simulink model "Day_08_Sliding_Mode_Control"  (R2024a)
settings: Solver=daessc  StartTime=0.0  StopTime=3  FixedStep=0.001  RelTol=1e-3
values from neighbouring files (symbols this model uses):
  C_theta = 3    [Day_08.m]
  C_x = 1    [Day_08.m]
  D0 = 2700    [Day_08.m]
  D1 = 2700    [Day_08.m]
  epsilon = 0.5    [Day_08.m]
  K = 100    [Day_08.m]
  L0 = 0.01    [Day_08.m]
  L1 = 0.14    [Day_08.m]
  lambda = 1    [Day_08.m]
  limit = .45    (= 0.45)    [Day_08.m]
  m = 3    [Day_08.m]
  M0 = L0*W0*T0*D0    (= 0.0027)    [Day_08.m]
  M1 = L1*W1*T1*D1    (= 0.0378)    [Day_08.m]
  T0 = 0.01    [Day_08.m]
  T1 = 0.01    [Day_08.m]
  W0 = 0.01    [Day_08.m]
  W1 = 0.01    [Day_08.m]
  x1_d = 0    [Day_08.m]
  x2_d = 0    [Day_08.m]
  x3_d = 0    [Day_08.m]
  x4_d = 0    [Day_08.m]
undefined symbols (not defined in the file or in its folder): X, Y, Z
libraries: sm_lib x14, nesl_utility x7
settings Model: Creator=mingeun  LastModifiedBy=mingeun
settings SolverCC: ZeroCrossAlgorithm=Adaptive
settings DataIOCC: ReturnWorkspaceOutputs=off
settings OptimizationCC: BlockReduction=off  DefaultParameterBehavior=Inlined  BufferReuse=off
settings DebuggingCC: IgnoredZcDiagnostic=none

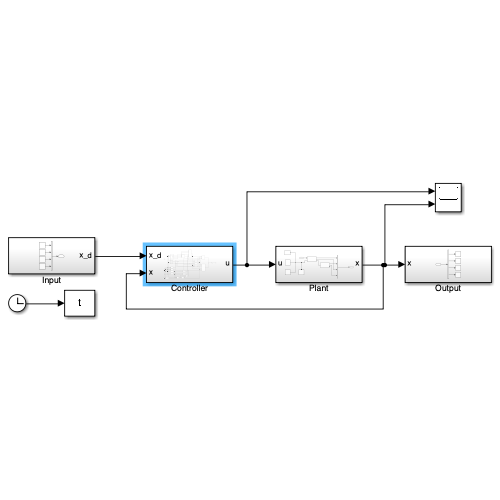
[thumbnail: Simulink's stored preview of the top-level diagram]
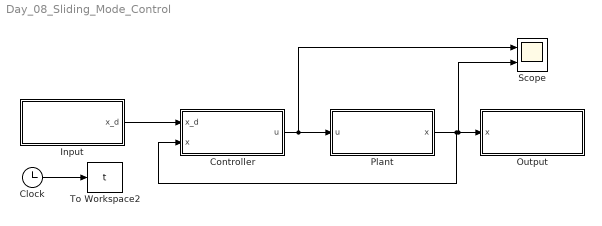
== system Day_08_Sliding_Mode_Control ==
  Clock : Clock
  Controller : Subsystem
  Input : Subsystem
  Output : Subsystem
  Plant : Subsystem
  Scope : Scope  NumInputPorts=2
  To Workspace2 : ToWorkspace  VariableName=t  SampleTime=-1
  wires:
  Clock/1 -> To Workspace2/1
  Input/1(x_d) -> Controller/1(x_d)
  Controller/1(u) -> Scope/1, Plant/1(u)
  Plant/1(x) -> Scope/2, Output/1(x), Controller/2(x)

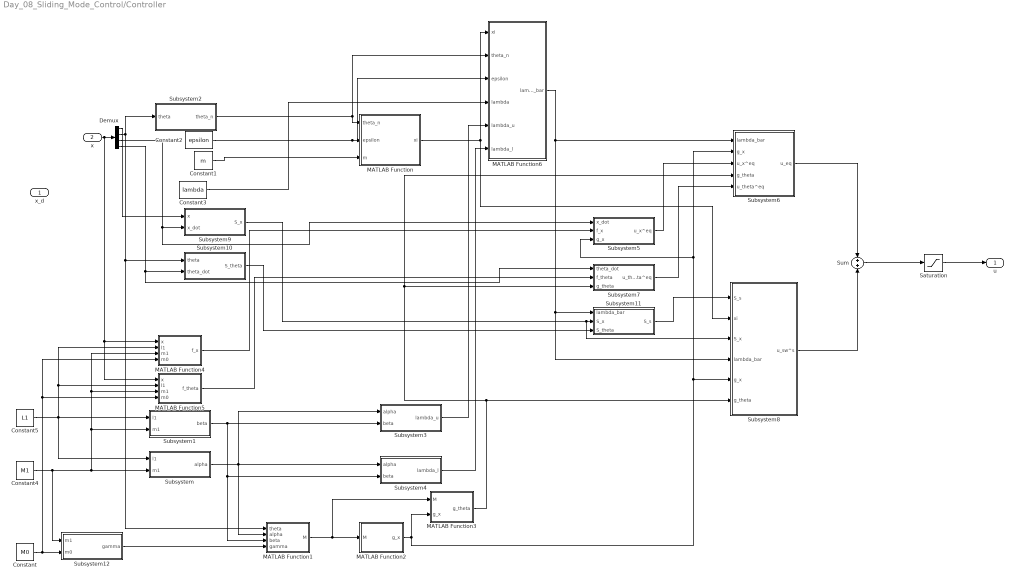
== system Day_08_Sliding_Mode_Control/Controller ==
  x_d : Inport
  x : Inport  Port=2
  Constant : Constant  Value=M0
  Constant1 : Constant  Value=m
  Constant2 : Constant  Value=epsilon
  Constant3 : Constant  Value=lambda
  Constant4 : Constant  Value=M1
  Constant5 : Constant  Value=L1
  Demux : Demux
  MATLAB Function : MATLAB Function  TreatAsAtomicUnit=on
  MATLAB Function1 : MATLAB Function  TreatAsAtomicUnit=on
  MATLAB Function2 : MATLAB Function  TreatAsAtomicUnit=on
  MATLAB Function3 : MATLAB Function  TreatAsAtomicUnit=on
  MATLAB Function4 : MATLAB Function  TreatAsAtomicUnit=on
  MATLAB Function5 : MATLAB Function  TreatAsAtomicUnit=on
  MATLAB Function6 : MATLAB Function  TreatAsAtomicUnit=on
  Saturation : Saturate  UpperLimit=limit  LowerLimit=-limit
  Subsystem : Subsystem
  Subsystem1 : Subsystem
  Subsystem10 : Subsystem
  Subsystem11 : Subsystem
  Subsystem12 : Subsystem
  Subsystem2 : Subsystem
  Subsystem3 : Subsystem
  Subsystem4 : Subsystem
  Subsystem5 : Subsystem
  Subsystem6 : Subsystem
  Subsystem7 : Subsystem
  Subsystem8 : Subsystem
  Subsystem9 : Subsystem
  Sum : Sum  Inputs=+|+
  u : Outport
  wires:
  Saturation/1 -> u/1
  x/1 -> Demux/1, MATLAB Function5/1(x), MATLAB Function4/1(x)
  Demux/2 -> Subsystem2/1(theta), Subsystem10/1(theta), MATLAB Function1/1(theta)
  Constant1/1 -> MATLAB Function/3(m)
  Constant2/1 -> MATLAB Function6/3(epsilon), MATLAB Function/2(epsilon)
  Constant5/1 -> Subsystem1/1(l1), Subsystem/1(l1), MATLAB Function5/2(l1), MATLAB Function4/2(l1)
  Constant4/1 -> Subsystem1/2(m1), MATLAB Function5/3(m1), MATLAB Function4/3(m1), Subsystem/2(m1), Subsystem12/1(m1)
  Subsystem/1(alpha) -> MATLAB Function1/2(alpha), Subsystem3/1(alpha), Subsystem4/1(alpha)
  Subsystem1/1(beta) -> MATLAB Function1/3(beta), Subsystem4/2(beta), Subsystem3/2(beta)
  Constant/1 -> MATLAB Function5/4(m0), MATLAB Function4/4(m0), Subsystem12/2(m0)
  MATLAB Function1/1(M) -> MATLAB Function3/1(M), MATLAB Function2/1(M)
  MATLAB Function2/1(g_x) -> Subsystem8/5(g_x), Subsystem6/2(g_x), Subsystem5/3(g_x), MATLAB Function3/2(g_x)
  Subsystem2/1(theta_n) -> MATLAB Function6/2(theta_n), MATLAB Function/1(theta_n)
  Constant3/1 -> MATLAB Function6/4(lambda)
  Subsystem3/1(lambda_u) -> MATLAB Function6/5(lambda_u)
  Subsystem4/1(lambda_l) -> MATLAB Function6/6(lambda_l)
  MATLAB Function3/1(g_theta) -> Subsystem7/3(g_theta), Subsystem6/4(g_theta), Subsystem8/6(g_theta)
  Demux/3 -> Subsystem9/2(x_dot), Subsystem5/1(x_dot)
  Demux/4 -> Subsystem7/1(theta_dot), Subsystem10/2(theta_dot)
  MATLAB Function4/1(f_x) -> Subsystem5/2(f_x)
  MATLAB Function5/1(f_theta) -> Subsystem7/2(f_theta)
  Subsystem7/1(u_theta^eq) -> Subsystem6/5(u_theta^eq)
  Subsystem5/1(u_x^eq) -> Subsystem6/3(u_x^eq)
  Demux/1 -> Subsystem9/1(x)
  Subsystem9/1(S_x) -> Subsystem8/3(S_x), Subsystem11/2(S_x)
  Subsystem10/1(S_theta) -> Subsystem11/3(S_theta)
  Subsystem11/1(S_s) -> Subsystem8/1(S_s)
  MATLAB Function/1(xi) -> MATLAB Function6/1(xi), Subsystem8/2(xi)
  MATLAB Function6/1(lambda_bar) -> Subsystem8/4(lambda_bar), Subsystem11/1(lambda_bar), Subsystem6/1(lambda_bar)
  Subsystem6/1(u_eq) -> Sum/1
  Subsystem8/1(u_sw^s) -> Sum/2
  Sum/1 -> Saturation/1
  Subsystem12/1(gamma) -> MATLAB Function1/4(gamma)

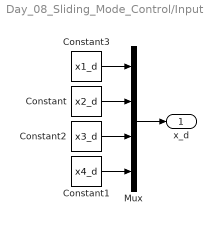
== system Day_08_Sliding_Mode_Control/Input ==
  Constant : Constant  Value=x2_d
  Constant1 : Constant  Value=x4_d
  Constant2 : Constant  Value=x3_d
  Constant3 : Constant  Value=x1_d
  Mux : Mux
  x_d : Outport
  wires:
  Mux/1 -> x_d/1
  Constant1/1 -> Mux/4
  Constant2/1 -> Mux/3
  Constant/1 -> Mux/2
  Constant3/1 -> Mux/1

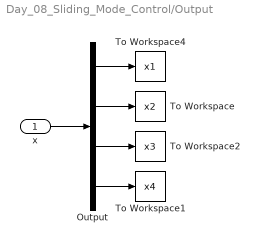
== system Day_08_Sliding_Mode_Control/Output ==
  x : Inport
  Output : Demux
  To Workspace : ToWorkspace  VariableName=x2  SampleTime=-1
  To Workspace1 : ToWorkspace  VariableName=x4  SampleTime=-1
  To Workspace2 : ToWorkspace  VariableName=x3  SampleTime=-1
  To Workspace4 : ToWorkspace  VariableName=x1  SampleTime=-1
  wires:
  Output/3 -> To Workspace2/1
  Output/4 -> To Workspace1/1
  Output/2 -> To Workspace/1
  Output/1 -> To Workspace4/1
  x/1 -> Output/1

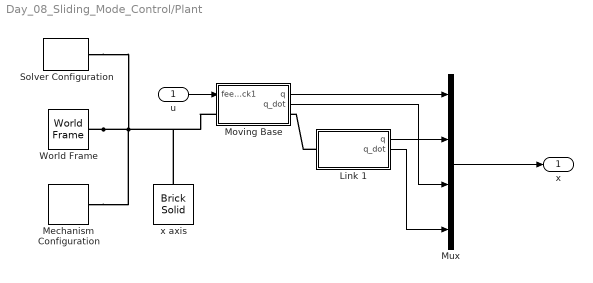
== system Day_08_Sliding_Mode_Control/Plant ==
  u : Inport
  Link 1 : Subsystem  mask{L=L1*100, W=W1*100, H=T1*100, rho=D1, rgb=[0.25 0.40 0.70], angle=150, F=0}
      mask prompts: L "Length (cm)"; W "Width (cm)"; H "Thickness (cm)"; rho "Density (kg/m^3)"; rgb "Color [R G B]"; angle "Initial Angle (degree)"; F "Disturbance [N]"
  Mechanism Configuration : sm_lib/Utilities/Mechanism Configuration  UniformGravity=Constant  GravityVector=[0 0 -9.80665]  GravityVectorUnits=m/s^2  LinearizationDelta=0.001  JointModeTransitionNonlinearIterations=2
  Moving Base : Subsystem  mask{L=L0*100, W=W0*100, H=T0*100, rho=D0, RGB=[0.8 0.45 0.0]}
      mask prompts: L "Length (cm)"; W "Width (cm)"; H "Thickness (cm)"; rho "Density (kg/m^3)"; RGB "Color [R G B]"
  Mux : Mux
  Solver Configuration : nesl_utility/Solver Configuration  PhysicalDomain=network_engine_domain  SubClassName=solver  LeftPortType=input  RightPortType=generic  Tones=[]  Harmonics=[]  SimulateNoise=off  Profile=off  UseLocalSampling=off  EnableSwitchedLinearOptims=on  FrequencyDomain=off  UseCCode=off  RelTol=0.001  AbsTol=0.001  MinStep=1e-09  ToWorkspace=off  RevertToSquareIcSolve=off  NumHomotopyIterations=100  PhasorMode=off  PhasorModeNumHarmonics=1  ConsistencySolver=NEWTON_XTOL_AFTER_FTOL  IndexReductionMethod=DerivativeReplacement  DoDC=off  ResidualTolerance=1e-09  ConsistencyTolSource=GLOBAL  ConsistencyAbsTol=0.001  ConsistencyRelTol=0.001  ConsistencyTolFactor=0.001  UseLocalSolver=off  LocalSolverChoice=NE_BACKWARD_EULER_ADVANCER  ResolveIndetEquations=on  FunctionEvalNumThread=1  LocalSolverSampleTime=0.001  DoFixedCost=off  MaxNonlinIter=3  MaxModeIter=2  ComputeImpulses=off  ImpulseIterations=2  LinearAlgebra=auto  LinearAlgebraNumThread=0  EquationFormulation=NE_TIME_EF  DelaysMemoryBudget=1024  AutomaticFiltering=on  FilteringTimeConstant=0.001  PartitionStorageMethod=AS_NEEDED  PartitionMemoryBudget=1024  PartitionMethod=ROBUST  MultibodyUseLocalSolver=off  MultibodyLocalSolverChoice=ODE1  MultibodyLocalSolverSampleTime=0.001
  World Frame : sm_lib/Frames and Transforms/World Frame
  x axis : sm_lib/Body Elements/Brick Solid  BrickDimensions=[1000 1 1]  BrickDimensionsUnits=mm  ExportEntireGeometry=off  InertiaType=CalculateFromGeometry  BasedOnType=Density  Density=1000  DensityUnits=kg/m^3  Mass=1  MassUnits=kg  CenterOfMass=[0 0 0]  CenterOfMassUnits=m  MomentsOfInertia=[1 1 1]  MomentsOfInertiaUnits=kg*m^2  ProductsOfInertia=[0 0 0]  ProductsOfInertiaUnits=kg*m^2  GraphicType=FromGeometry  MarkerShape=Sphere  MarkerSize=10  GraphicVisPropType=SimpleVisualProperties  GraphicDiffuseColor=[0.0 0.0 0.0]  GraphicOpacity=1  GraphicSpecularColor=[0.5 0.5 0.5 1.0]  GraphicAmbientColor=[0.15 0.15 0.15 1.0]  GraphicEmissiveColor=[0.0 0.0 0.0 1.0]  GraphicShininess=75  DoExposeReferenceFrame=on  SerializedFrames=<Frames/>
  x : Outport
  wires:
  Moving Base/1(q) -> Mux/1
  Link 1/1(q) -> Mux/2
  u/1 -> Moving Base/1(feedback1)
  Link 1/2(q_dot) -> Mux/4
  Moving Base/2(q_dot) -> Mux/3
  Mux/1 -> x/1
  connections:
  World Frame/RConn1 -- Solver Configuration/RConn1 -- Moving Base/LConn1 -- x axis/RConn1 -- Mechanism Configuration/RConn1
  Link 1/LConn1 -- Moving Base/RConn1

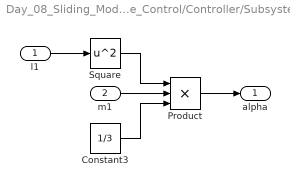
== system Day_08_Sliding_Mode_Control/Controller/Subsystem ==
  l1 : Inport
  m1 : Inport  Port=2
  Constant3 : Constant  Value=1/3
  Product : Product  Inputs=3
  Square : Math  Operator=square
  alpha : Outport
  wires:
  Product/1 -> alpha/1
  m1/1 -> Product/2
  Constant3/1 -> Product/3
  Square/1 -> Product/1
  l1/1 -> Square/1

== system Day_08_Sliding_Mode_Control/Controller/Subsystem1 ==
  l1 : Inport
  m1 : Inport  Port=2
  Constant7 : Constant  Value=1/2
  Product1 : Product  Inputs=3
  beta : Outport
  wires:
  Constant7/1 -> Product1/3
  Product1/1 -> beta/1
  l1/1 -> Product1/1
  m1/1 -> Product1/2

== system Day_08_Sliding_Mode_Control/Controller/Subsystem10 ==
  theta : Inport
  theta_dot : Inport  Port=2
  Gain : Gain  Gain=C_theta
  Sum : Sum  Inputs=|++
  S_theta : Outport
  wires:
  Sum/1 -> S_theta/1
  theta_dot/1 -> Sum/2
  Gain/1 -> Sum/1
  theta/1 -> Gain/1

== system Day_08_Sliding_Mode_Control/Controller/Subsystem11 ==
  lambda_bar : Inport
  S_x : Inport  Port=2
  S_theta : Inport  Port=3
  Product : Product
  Sum : Sum  Inputs=|++
  S_s : Outport
  wires:
  S_theta/1 -> Sum/2
  Product/1 -> Sum/1
  S_x/1 -> Product/2
  Sum/1 -> S_s/1
  lambda_bar/1 -> Product/1

== system Day_08_Sliding_Mode_Control/Controller/Subsystem12 ==
  m1 : Inport
  m0 : Inport  Port=2
  Sum : Sum  Inputs=|++
  gamma : Outport
  wires:
  Sum/1 -> gamma/1
  m0/1 -> Sum/2
  m1/1 -> Sum/1

== system Day_08_Sliding_Mode_Control/Controller/Subsystem2 ==
  theta : Inport
  Abs : Abs  SaturateOnIntegerOverflow=off
  Constant : Constant  Value=pi/2
  Sum : Sum  Inputs=|+-
  theta_n : Outport
  wires:
  Sum/1 -> theta_n/1
  Constant/1 -> Sum/2
  Abs/1 -> Sum/1
  theta/1 -> Abs/1

== system Day_08_Sliding_Mode_Control/Controller/Subsystem3 ==
  alpha : Inport
  beta : Inport  Port=2
  Divide : Product  Inputs=/**
  theta_u^star : Constant  Value=pi/2-epsilon
  lambda_u : Outport
  wires:
  Divide/1 -> lambda_u/1
  theta_u^star/1 -> Divide/3
  beta/1 -> Divide/2
  alpha/1 -> Divide/1

== system Day_08_Sliding_Mode_Control/Controller/Subsystem4 ==
  alpha : Inport
  beta : Inport  Port=2
  Divide : Product  Inputs=/**
  theta_l^star1 : Constant  Value=pi/2+epsilon
  lambda_l : Outport
  wires:
  Divide/1 -> lambda_l/1
  beta/1 -> Divide/2
  alpha/1 -> Divide/1
  theta_l^star1/1 -> Divide/3

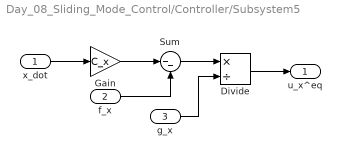
== system Day_08_Sliding_Mode_Control/Controller/Subsystem5 ==
  x_dot : Inport
  f_x : Inport  Port=2
  g_x : Inport  Port=3
  Divide : Product  Inputs=*/
  Gain : Gain  Gain=C_x
  Sum : Sum  Inputs=|--
  u_x^eq : Outport
  wires:
  Divide/1 -> u_x^eq/1
  g_x/1 -> Divide/2
  f_x/1 -> Sum/2
  Sum/1 -> Divide/1
  Gain/1 -> Sum/1
  x_dot/1 -> Gain/1

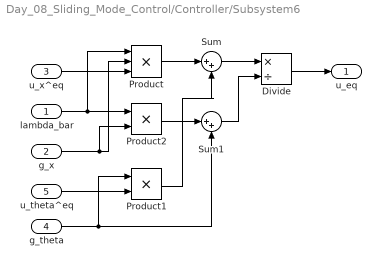
== system Day_08_Sliding_Mode_Control/Controller/Subsystem6 ==
  lambda_bar : Inport
  g_x : Inport  Port=2
  u_x^eq : Inport  Port=3
  g_theta : Inport  Port=4
  u_theta^eq : Inport  Port=5
  Divide : Product  Inputs=*/
  Product : Product  Inputs=3
  Product1 : Product
  Product2 : Product
  Sum : Sum  Inputs=|++
  Sum1 : Sum  Inputs=|++
  u_eq : Outport
  wires:
  Divide/1 -> u_eq/1
  Sum/1 -> Divide/1
  Sum1/1 -> Divide/2
  Product1/1 -> Sum/2
  Product/1 -> Sum/1
  g_theta/1 -> Product1/1, Sum1/2
  g_x/1 -> Product2/2, Product/2
  lambda_bar/1 -> Product2/1, Product/1
  u_theta^eq/1 -> Product1/2
  Product2/1 -> Sum1/1
  u_x^eq/1 -> Product/3

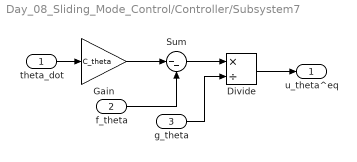
== system Day_08_Sliding_Mode_Control/Controller/Subsystem7 ==
  theta_dot : Inport
  f_theta : Inport  Port=2
  g_theta : Inport  Port=3
  Divide : Product  Inputs=*/
  Gain : Gain  Gain=C_theta
  Sum : Sum  Inputs=|--
  u_theta^eq : Outport
  wires:
  g_theta/1 -> Divide/2
  Sum/1 -> Divide/1
  Divide/1 -> u_theta^eq/1
  f_theta/1 -> Sum/2
  Gain/1 -> Sum/1
  theta_dot/1 -> Gain/1

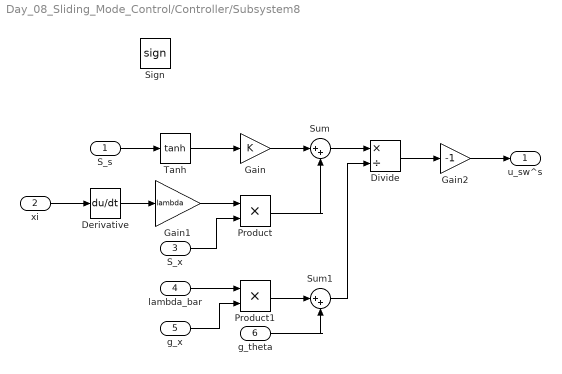
== system Day_08_Sliding_Mode_Control/Controller/Subsystem8 ==
  S_s : Inport
  xi : Inport  Port=2
  S_x : Inport  Port=3
  lambda_bar : Inport  Port=4
  g_x : Inport  Port=5
  g_theta : Inport  Port=6
  Derivative : Derivative
  Divide : Product  Inputs=*/
  Gain : Gain  Gain=K
  Gain1 : Gain  Gain=lambda
  Gain2 : Gain  Gain=-1
  Product : Product
  Product1 : Product
  Sign : Signum
  Sum : Sum  Inputs=|++
  Sum1 : Sum  Inputs=|++
  Tanh : Trigonometry  Operator=tanh
  u_sw^s : Outport
  wires:
  Gain2/1 -> u_sw^s/1
  Sum1/1 -> Divide/2
  Sum/1 -> Divide/1
  g_theta/1 -> Sum1/2
  xi/1 -> Derivative/1
  lambda_bar/1 -> Product1/1
  Product1/1 -> Sum1/1
  Product/1 -> Sum/2
  g_x/1 -> Product1/2
  S_x/1 -> Product/2
  Gain/1 -> Sum/1
  Gain1/1 -> Product/1
  Divide/1 -> Gain2/1
  S_s/1 -> Tanh/1
  Tanh/1 -> Gain/1
  Derivative/1 -> Gain1/1

== system Day_08_Sliding_Mode_Control/Controller/Subsystem9 ==
  x : Inport
  x_dot : Inport  Port=2
  Gain : Gain  Gain=C_x
  Sum : Sum  Inputs=|++
  S_x : Outport
  wires:
  x_dot/1 -> Sum/2
  Sum/1 -> S_x/1
  Gain/1 -> Sum/1
  x/1 -> Gain/1

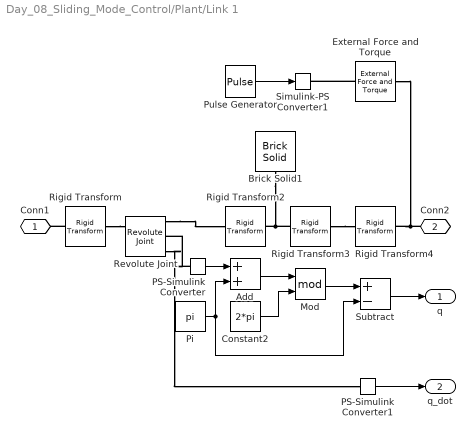
== system Day_08_Sliding_Mode_Control/Plant/Link 1 ==
  Add : Sum
  Brick Solid1 : sm_lib/Body Elements/Brick Solid  BrickDimensions=[L W H]  BrickDimensionsUnits=cm  ExportEntireGeometry=off  InertiaType=CalculateFromGeometry  BasedOnType=Density  Density=rho  DensityUnits=kg/m^3  Mass=1  MassUnits=kg  CenterOfMass=[0 0 0]  CenterOfMassUnits=m  MomentsOfInertia=[1 1 1]  MomentsOfInertiaUnits=kg*m^2  ProductsOfInertia=[0 0 0]  ProductsOfInertiaUnits=kg*m^2  GraphicType=FromGeometry  MarkerShape=Sphere  MarkerSize=10  GraphicVisPropType=SimpleVisualProperties  GraphicDiffuseColor=rgb  GraphicOpacity=1  GraphicSpecularColor=[0.5 0.5 0.5 1.0]  GraphicAmbientColor=[0.15 0.15 0.15 1.0]  GraphicEmissiveColor=[0.0 0.0 0.0 1.0]  GraphicShininess=75  DoExposeReferenceFrame=on  SerializedFrames=<Frames/>
  Constant2 : Constant  Value=2*pi
  External Force and Torque : sm_lib/Forces and Torques/External Force and Torque  EnableForceX=on  EnableForceY=off  EnableForceZ=off  EnableForce=off  ForceResolutionFrame=World  EnableTorqueX=off  EnableTorqueY=off  EnableTorqueZ=off  EnableTorque=off  TorqueResolutionFrame=World
  Mod : Math  Operator=mod  OutputSignalType=real
  PS-Simulink Converter : nesl_utility/PS-Simulink Converter  PhysicalDomain=network_engine_domain  SubClassName=ps_output  LeftPortType=input  RightPortType=output  PseudoPeriodic=off  Frequencies=[]  VectorFormat=inherit  Unit=inherit  AffineConversion=off
  PS-Simulink Converter1 : nesl_utility/PS-Simulink Converter  PhysicalDomain=network_engine_domain  SubClassName=ps_output  LeftPortType=input  RightPortType=output  PseudoPeriodic=off  Frequencies=[]  VectorFormat=inherit  Unit=inherit  AffineConversion=off
  Pi : Constant  Value=pi  OutDataTypeStr=Inherit: Inherit via back propagation
  Pulse Generator : DiscretePulseGenerator  PulseType=Time based  Amplitude=F  Period=1000000  PulseWidth=1/1000000  PhaseDelay=0.25
  Revolute Joint : sm_lib/Joints/Revolute Joint  JointMode=Normal  CompositeWrenchDir=FollowerOnBase  CompositeWrenchFrame=BaseFrame  SenseConstraintForce=off  SenseConstraintTorque=off  SenseTotalForce=off  SenseTotalTorque=off  PositionTargetSpecify=on  PositionTargetPriority=High  PositionTargetValue=angle  PositionTargetValueUnits=deg  VelocityTargetSpecify=off  VelocityTargetPriority=High  VelocityTargetValue=0  VelocityTargetValueUnits=deg/s  EquilibriumPosition=0  EquilibriumPositionUnits=deg  SpringStiffness=0  SpringStiffnessUnits=N*m/deg  DampingCoefficient=0  DampingCoefficientUnits=N*m/(deg/s)  LowerLimitSpecify=off  LowerLimitBound=-90  LowerLimitBoundUnits=deg  LowerLimitStiffness=1e4  LowerLimitStiffnessUnits=N*m/deg  LowerLimitDamping=10  LowerLimitDampingUnits=N*m/(deg/s)  LowerLimitTransitionRegionWidth=0.1  LowerLimitTransitionRegionWidthUnits=deg  UpperLimitSpecify=off  UpperLimitBound=90  UpperLimitBoundUnits=deg  UpperLimitStiffness=1e4  UpperLimitStiffnessUnits=N*m/deg  UpperLimitDamping=10  UpperLimitDampingUnits=N*m/(deg/s)  UpperLimitTransitionRegionWidth=0.1  UpperLimitTransitionRegionWidthUnits=deg  TorqueActuationMode=InputTorque  MotionActuationMode=ComputedMotion  SensePosition=on  SenseVelocity=on  SenseAcceleration=off  SenseTorqueForce=off  SenseLowerLimitTorqueForce=off  SenseUpperLimitTorqueForce=off
  Rigid Transform : sm_lib/Frames and Transforms/Rigid Transform  RotationMethod=RotationMatrix  FollAlignAxisA=+X  BaseAlignAxisA=+Y  FollAlignAxisB=+Y  BaseAlignAxisB=+Z  RotationStandardAxis=+X  RotationAngle=90  RotationAngleUnits=deg  RotationArbitraryAxis=[0 0 1]  RotationSequenceAxes=FollowerAxes  RotationSequence=XYX  RotationSequenceAngles=[0 0 0]  RotationSequenceAnglesUnits=deg  RotationMatrix=[0 0 1; 1 0 0; 0 1 0]  Quaternion=[1 0 0 0]  TranslationMethod=None  TranslationCartesianOffset=[0 0 0]  TranslationCartesianOffsetUnits=m  TranslationStandardAxis=+Z  TranslationStandardOffset=0  TranslationStandardOffsetUnits=m  TranslationROffset=0  TranslationROffsetUnits=m  TranslationThetaOffset=0  TranslationThetaOffsetUnits=deg  TranslationZOffset=0  TranslationZOffsetUnits=m
  Rigid Transform2 : sm_lib/Frames and Transforms/Rigid Transform  RotationMethod=None  FollAlignAxisA=+X  BaseAlignAxisA=+Y  FollAlignAxisB=+Y  BaseAlignAxisB=+Z  RotationStandardAxis=+Z  RotationAngle=0  RotationAngleUnits=deg  RotationArbitraryAxis=[0 0 1]  RotationSequenceAxes=FollowerAxes  RotationSequence=XYX  RotationSequenceAngles=[0 0 0]  RotationSequenceAnglesUnits=deg  RotationMatrix=[1 0 0;0 1 0;0 0 1]  Quaternion=[1 0 0 0]  TranslationMethod=StandardAxis  TranslationCartesianOffset=[0 0 0]  TranslationCartesianOffsetUnits=m  TranslationStandardAxis=-X  TranslationStandardOffset=L/2  TranslationStandardOffsetUnits=cm  TranslationROffset=0  TranslationROffsetUnits=m  TranslationThetaOffset=0  TranslationThetaOffsetUnits=deg  TranslationZOffset=0  TranslationZOffsetUnits=m
  Rigid Transform3 : sm_lib/Frames and Transforms/Rigid Transform  RotationMethod=None  FollAlignAxisA=+X  BaseAlignAxisA=+Y  FollAlignAxisB=+Y  BaseAlignAxisB=+Z  RotationStandardAxis=+Z  RotationAngle=0  RotationAngleUnits=deg  RotationArbitraryAxis=[0 0 1]  RotationSequenceAxes=FollowerAxes  RotationSequence=XYX  RotationSequenceAngles=[0 0 0]  RotationSequenceAnglesUnits=deg  RotationMatrix=[1 0 0;0 1 0;0 0 1]  Quaternion=[1 0 0 0]  TranslationMethod=StandardAxis  TranslationCartesianOffset=[0 0 0]  TranslationCartesianOffsetUnits=m  TranslationStandardAxis=-X  TranslationStandardOffset=L/2  TranslationStandardOffsetUnits=cm  TranslationROffset=0  TranslationROffsetUnits=m  TranslationThetaOffset=0  TranslationThetaOffsetUnits=deg  TranslationZOffset=0  TranslationZOffsetUnits=m
  Rigid Transform4 : sm_lib/Frames and Transforms/Rigid Transform  RotationMethod=None  FollAlignAxisA=+X  BaseAlignAxisA=+Y  FollAlignAxisB=+Y  BaseAlignAxisB=+Z  RotationStandardAxis=+Z  RotationAngle=0  RotationAngleUnits=deg  RotationArbitraryAxis=[0 0 1]  RotationSequenceAxes=FollowerAxes  RotationSequence=XYX  RotationSequenceAngles=[0 0 0]  RotationSequenceAnglesUnits=deg  RotationMatrix=[1 0 0; 0 0 1; 0 -1 0]  Quaternion=[1 0 0 0]  TranslationMethod=StandardAxis  TranslationCartesianOffset=[0 0 0]  TranslationCartesianOffsetUnits=m  TranslationStandardAxis=+X  TranslationStandardOffset=L  TranslationStandardOffsetUnits=cm  TranslationROffset=0  TranslationROffsetUnits=m  TranslationThetaOffset=0  TranslationThetaOffsetUnits=deg  TranslationZOffset=0  TranslationZOffsetUnits=m
  Simulink-PS Converter1 : nesl_utility/Simulink-PS Converter  PhysicalDomain=network_engine_domain  SubClassName=ps_input  LeftPortType=input  RightPortType=output  PseudoPeriodic=off  Frequencies=[]  NoiseDistribution=none  NoiseParameters=[]  Unit=1  AffineConversion=off  FilteringAndDerivatives=provide  SimscapeFilterOrder=1  InputFilterTimeConstant=0.001  UdotUserProvided=0
  Subtract : Sum  Inputs=+-
  Conn1 : PMIOPort  Side=Left
  Conn2 : PMIOPort  Port=2  Side=Right
  q : Outport
  q_dot : Outport  Port=2
  wires:
  Pulse Generator/1 -> Simulink-PS Converter1/1
  Mod/1 -> Subtract/1
  Constant2/1 -> Mod/2
  Pi/1 -> Subtract/2, Add/2
  PS-Simulink Converter/1 -> Add/1
  Add/1 -> Mod/1
  Subtract/1 -> q/1
  PS-Simulink Converter1/1 -> q_dot/1
  connections:
  PS-Simulink Converter/LConn1 -- Revolute Joint/RConn2
  Rigid Transform3/RConn1 -- Rigid Transform4/LConn1
  Rigid Transform/LConn1 -- Revolute Joint/LConn1
  Rigid Transform3/LConn1 -- Brick Solid1/RConn1 -- Rigid Transform2/LConn1
  Conn2/RConn1 -- External Force and Torque/RConn1 -- Rigid Transform4/RConn1
  Rigid Transform/RConn1 -- Conn1/RConn1
  Revolute Joint/RConn1 -- Rigid Transform2/RConn1
  External Force and Torque/LConn1 -- Simulink-PS Converter1/RConn1
  Revolute Joint/RConn3 -- PS-Simulink Converter1/LConn1

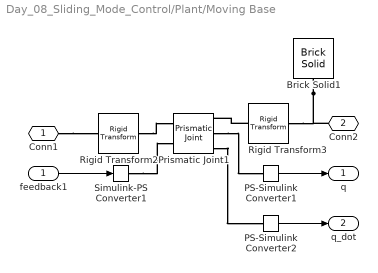
== system Day_08_Sliding_Mode_Control/Plant/Moving Base ==
  feedback1 : Inport
  Brick Solid1 : sm_lib/Body Elements/Brick Solid  BrickDimensions=[L W H]  BrickDimensionsUnits=cm  ExportEntireGeometry=off  InertiaType=CalculateFromGeometry  BasedOnType=Density  Density=rho  DensityUnits=kg/m^3  Mass=1  MassUnits=kg  CenterOfMass=[0 0 0]  CenterOfMassUnits=m  MomentsOfInertia=[1 1 1]  MomentsOfInertiaUnits=kg*m^2  ProductsOfInertia=[0 0 0]  ProductsOfInertiaUnits=kg*m^2  GraphicType=FromGeometry  MarkerShape=Sphere  MarkerSize=10  GraphicVisPropType=SimpleVisualProperties  GraphicDiffuseColor=RGB  GraphicOpacity=1  GraphicSpecularColor=[0.5 0.5 0.5 1.0]  GraphicAmbientColor=[0.15 0.15 0.15 1.0]  GraphicEmissiveColor=[0.0 0.0 0.0 1.0]  GraphicShininess=75  DoExposeReferenceFrame=on  SerializedFrames=<Frames/>
  PS-Simulink Converter1 : nesl_utility/PS-Simulink Converter  PhysicalDomain=network_engine_domain  SubClassName=ps_output  LeftPortType=input  RightPortType=output  PseudoPeriodic=off  Frequencies=[]  VectorFormat=inherit  Unit=inherit  AffineConversion=off
  PS-Simulink Converter2 : nesl_utility/PS-Simulink Converter  PhysicalDomain=network_engine_domain  SubClassName=ps_output  LeftPortType=input  RightPortType=output  PseudoPeriodic=off  Frequencies=[]  VectorFormat=inherit  Unit=inherit  AffineConversion=off
  Prismatic Joint1 : sm_lib/Joints/Prismatic Joint  JointMode=Normal  CompositeWrenchDir=FollowerOnBase  CompositeWrenchFrame=BaseFrame  SenseConstraintForce=off  SenseConstraintTorque=off  SenseTotalForce=off  SenseTotalTorque=off  PositionTargetSpecify=off  PositionTargetPriority=High  PositionTargetValue=0  PositionTargetValueUnits=m  VelocityTargetSpecify=off  VelocityTargetPriority=High  VelocityTargetValue=0  VelocityTargetValueUnits=m/s  EquilibriumPosition=0  EquilibriumPositionUnits=m  SpringStiffness=0  SpringStiffnessUnits=N/m  DampingCoefficient=0  DampingCoefficientUnits=N/(m/s)  LowerLimitSpecify=off  LowerLimitBound=-1  LowerLimitBoundUnits=m  LowerLimitStiffness=1e6  LowerLimitStiffnessUnits=N/m  LowerLimitDamping=1e3  LowerLimitDampingUnits=N/(m/s)  LowerLimitTransitionRegionWidth=1e-4  LowerLimitTransitionRegionWidthUnits=m  UpperLimitSpecify=off  UpperLimitBound=1  UpperLimitBoundUnits=m  UpperLimitStiffness=1e6  UpperLimitStiffnessUnits=N/m  UpperLimitDamping=1e3  UpperLimitDampingUnits=N/(m/s)  UpperLimitTransitionRegionWidth=1e-4  UpperLimitTransitionRegionWidthUnits=m  TorqueActuationMode=InputTorque  MotionActuationMode=ComputedMotion  SensePosition=on  SenseVelocity=on  SenseAcceleration=off  SenseTorqueForce=off  SenseLowerLimitTorqueForce=off  SenseUpperLimitTorqueForce=off
  Rigid Transform2 : sm_lib/Frames and Transforms/Rigid Transform  RotationMethod=StandardAxis  FollAlignAxisA=+X  BaseAlignAxisA=+Y  FollAlignAxisB=+Y  BaseAlignAxisB=+Z  RotationStandardAxis=+Y  RotationAngle=90  RotationAngleUnits=deg  RotationArbitraryAxis=[0 0 1]  RotationSequenceAxes=FollowerAxes  RotationSequence=XYX  RotationSequenceAngles=[0 0 0]  RotationSequenceAnglesUnits=deg  RotationMatrix=[1 0 0;0 1 0;0 0 1]  Quaternion=[1 0 0 0]  TranslationMethod=None  TranslationCartesianOffset=[0 0 0]  TranslationCartesianOffsetUnits=m  TranslationStandardAxis=+Z  TranslationStandardOffset=0  TranslationStandardOffsetUnits=m  TranslationROffset=0  TranslationROffsetUnits=m  TranslationThetaOffset=0  TranslationThetaOffsetUnits=deg  TranslationZOffset=0  TranslationZOffsetUnits=m
  Rigid Transform3 : sm_lib/Frames and Transforms/Rigid Transform  RotationMethod=StandardAxis  FollAlignAxisA=+X  BaseAlignAxisA=+Y  FollAlignAxisB=+Y  BaseAlignAxisB=+Z  RotationStandardAxis=+Y  RotationAngle=90  RotationAngleUnits=deg  RotationArbitraryAxis=[0 0 1]  RotationSequenceAxes=FollowerAxes  RotationSequence=XYX  RotationSequenceAngles=[0 0 0]  RotationSequenceAnglesUnits=deg  RotationMatrix=[1 0 0;0 1 0;0 0 1]  Quaternion=[1 0 0 0]  TranslationMethod=None  TranslationCartesianOffset=[0 0 0]  TranslationCartesianOffsetUnits=m  TranslationStandardAxis=+Z  TranslationStandardOffset=0  TranslationStandardOffsetUnits=m  TranslationROffset=0  TranslationROffsetUnits=m  TranslationThetaOffset=0  TranslationThetaOffsetUnits=deg  TranslationZOffset=0  TranslationZOffsetUnits=m
  Simulink-PS Converter1 : nesl_utility/Simulink-PS Converter  PhysicalDomain=network_engine_domain  SubClassName=ps_input  LeftPortType=input  RightPortType=output  PseudoPeriodic=off  Frequencies=[]  NoiseDistribution=none  NoiseParameters=[]  Unit=1  AffineConversion=off  FilteringAndDerivatives=provide  SimscapeFilterOrder=1  InputFilterTimeConstant=0.001  UdotUserProvided=0
  Conn1 : PMIOPort  Side=Left
  Conn2 : PMIOPort  Port=2  Side=Right
  q : Outport
  q_dot : Outport  Port=2
  wires:
  feedback1/1 -> Simulink-PS Converter1/1
  PS-Simulink Converter1/1 -> q/1
  PS-Simulink Converter2/1 -> q_dot/1
  connections:
  Brick Solid1/RConn1 -- Conn2/RConn1 -- Rigid Transform3/LConn1
  Rigid Transform2/RConn1 -- Prismatic Joint1/LConn1
  Prismatic Joint1/RConn2 -- PS-Simulink Converter1/LConn1
  Simulink-PS Converter1/RConn1 -- Prismatic Joint1/LConn2
  Conn1/RConn1 -- Rigid Transform2/LConn1
  Rigid Transform3/RConn1 -- Prismatic Joint1/RConn1
  Prismatic Joint1/RConn3 -- PS-Simulink Converter2/LConn1

== matlab function Day_08_Sliding_Mode_Control/Controller/MATLAB Function1 ==
  data: theta input; alpha input; beta input; M output; gamma input
function M = fcn(theta, alpha, beta, gamma)

M = [gamma, beta*cos(theta);
     beta*cos(theta), alpha];

== matlab function Day_08_Sliding_Mode_Control/Controller/MATLAB Function ==
  data: theta_n input; epsilon input; xi output; m input
function xi = calculateLambdaBar(theta_n, epsilon, m)
    % This function calculates the sum for the function N_m(z)
    % Inputs:
    %   theta_n - the input variable theta_n (scalar or vector)
    %   m - the order of factorial in the denominator (scalar)
    
    n = m + 1;
    Delta = (2/n)*epsilon;

    xi = 0; % Initialize the output
    for k = 0:n
        % Calculate the combination term binomial coefficient
        comb_nk = nchoosek(n, k);
        
        % Calculate the term in the brackets
        term = theta_n + (n/2 - k) * Delta;
        
        % Update the sum for N_m(z)
        xi = xi + ((-1)^k / factorial(m)) * comb_nk * term;
    end
end

== matlab function Day_08_Sliding_Mode_Control/Controller/MATLAB Function2 ==
  data: g_x output; M input
function g_x = fcn(M)

g_x = M(2, 2)/det(M);

== matlab function Day_08_Sliding_Mode_Control/Controller/MATLAB Function3 ==
  data: M input; g_theta output; g_x input
function g_theta = fcn(M, g_x)

g_theta = -M(2, 1)*g_x/M(2, 2);

== matlab function Day_08_Sliding_Mode_Control/Controller/MATLAB Function4 ==
  data: x input; l1 input; m1 input; m0 input; f_x output
function f_x = fcn(x, l1, m1, m0)

x1 = x(1);
x2 = x(2);
x3 = x(3);
x4 = x(4);
g = 9.81;

% f_x = (m1*sin(x2)*(3*g*cos(x2) - 2*l1*x4^2))/(4*m0 + 4*m1 - 3*m1*cos(x2)^2);

f_x = -(m1*sin(x2)*(3*g*cos(x2) - 2*l1*x4^2))/(4*m0 + 4*m1 - 3*m1*cos(x2)^2);

== matlab function Day_08_Sliding_Mode_Control/Controller/MATLAB Function5 ==
  data: x input; l1 input; m1 input; f_theta output; m0 input
function f_theta = fcn(x, l1, m1, m0)

x1 = x(1);
x2 = x(2);
x3 = x(3);
x4 = x(4);
g = 9.81;

% f_theta = (3*sin(x2)*(2*g*m0 + 2*g*m1 - l1*m1*cos(x2)*x4^2))/(l1*(4*m0 + 4*m1 - 3*m1*cos(x2)^2));

f_theta = (3*sin(x2)*(2*g*m0 + 2*g*m1 - l1*m1*cos(x2)*x4^2))/(l1*(4*m0 + 4*m1 - 3*m1*cos(x2)^2));

== matlab function Day_08_Sliding_Mode_Control/Controller/MATLAB Function6 ==
  data: xi input; lambda_bar output; theta_n input; epsilon input; lambda input; lambda_u input; lambda_l input
function lambda_bar = fcn(xi, theta_n, epsilon,lambda, lambda_u, lambda_l)

lambda_bar = lambda*(xi-1)*sign(theta_n);
if theta_n > epsilon
    lambda_bar = lambda_l;
elseif theta_n < -epsilon
    lambda_bar = lambda_u;
end
